simulink model "SSC"  (R2018b)
settings: Solver=ode23tb  StartTime=0.0  StopTime=5  RelTol=1e-3  EnableMultiTasking=on
values from neighbouring files (symbols this model uses):
  simSwitchingFrequency = 500.0    [SSC.sldd]
libraries: powerlib x15, powerlib_meascontrol x4, raspberrypilib x2, simulink x1, dspsrcs4 x1
settings Model: DataDictionary=SSC.sldd  SimulationMode=accelerator  Creator=guido  LastModifiedBy=guido
settings SolverCC: PositivePriorityOrder=on
settings OptimizationCC: EnhancedBackFolding=on  PassReuseOutputArgsAs=Individual arguments  EfficientMapNaN2IntZero=off  MaxStackSize=64  OptimizeBlockOrder=speed  DifferentSizesBufferReuse=on
settings DebuggingCC: ParameterTunabilityLossMsg=error
settings HardwareCC: ProdBitPerPointer=32  ProdBitPerSizeT=32  ProdBitPerPtrDiffT=32  ProdLargestAtomicInteger=Long  ProdLargestAtomicFloat=Double  ProdWordSize=32  ProdHWDeviceType=ARM Compatible->ARM Cortex  TargetBitPerPointer=64  TargetBitPerSizeT=64  TargetBitPerPtrDiffT=64  TargetLargestAtomicInteger=Long  TargetLongLongMode=on  TargetIntDivRoundTo=Zero  TargetEndianess=LittleEndian  TargetWordSize=64  TargetHWDeviceType=MATLAB Host  ProdEqTarget=off  UseEmbeddedCoderFeatures=off
settings SFSimCC: MATLABDynamicMemAlloc=off
settings CodeAppCC: MaxIdLength=128
settings GRTTargetCC: TargetLangStandard=C89/C90 (ANSI)  CombineOutputUpdateFcns=off  GRTInterface=on

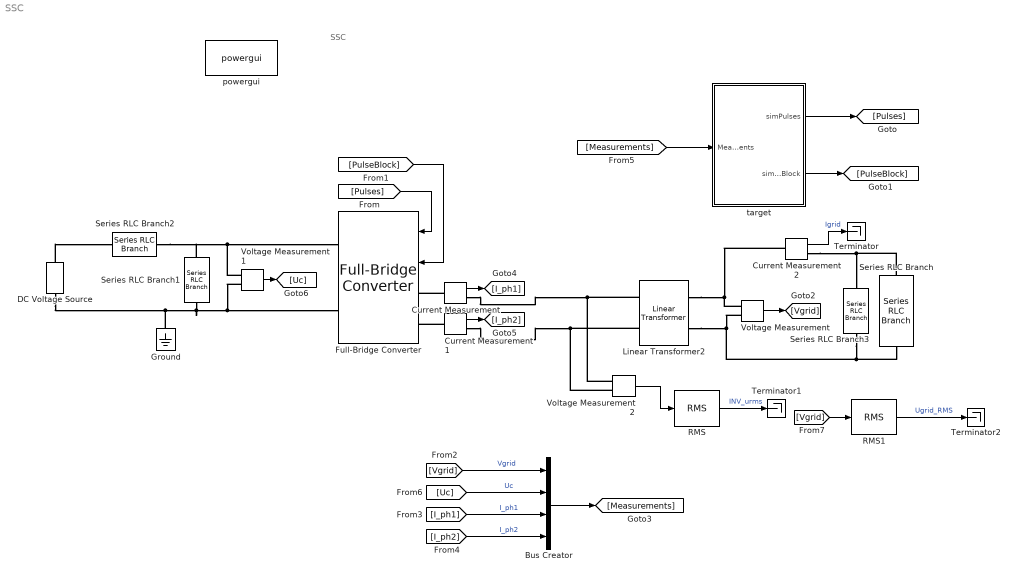
== system SSC ==
  note: SSC
  Bus Creator : BusCreator  Inputs=4  OutDataTypeStr=Bus: MeasurementsBus
  Current Measurement : powerlib/Measurements/Current Measurement  PhasorSimulation=off  OutputType=Complex  PSBequivalent=0
  Current Measurement1 : powerlib/Measurements/Current Measurement  PhasorSimulation=off  OutputType=Complex  PSBequivalent=0
  Current Measurement2 : powerlib/Measurements/Current Measurement  PhasorSimulation=off  OutputType=Complex  PSBequivalent=0
  DC Voltage Source : powerlib/Electrical Sources/DC Voltage Source  Amplitude=24  Measurements=None
  Full-Bridge Converter : powerlib/Power Electronics/Full-Bridge Converter  ModelType=Switching devices  Ron=1e-3  Rs=1e6  Cs=inf  Vforward=[0,0]  Ron_Diode=1e-3  Rs_Diode=1e6  Cs_Diode=inf  Vf_Diode=1e-3  Rs_CurrentSource=inf
      settings: SourceProductName=Simscape Power Systems  SourceProductBaseCode=PS
  Ground : powerlib/Elements/Ground  LConnTagsString=a
  Linear Transformer2 : powerlib/Elements/Linear Transformer  UNITS=pu  NominalPower=[ 1e3 50 ]  winding1="[ 12  0.002  0.08 ]"  winding2="[ 230  0.002  0.08 ]"  ThreeWindings=off  winding3=[ 315e3 0.002 0.08 ]  RmLm=[ 500 500 ]  Measurements=None  DataType=off
  RMS : powerlib_meascontrol/Measurements/RMS  TrueRMS=on  Freq=50  RMSInit=0  Ts=0
  RMS1 : powerlib_meascontrol/Measurements/RMS  TrueRMS=on  Freq=50  RMSInit=0  Ts=0
  Series RLC Branch : powerlib/Elements/Series RLC Branch  LConnTagsString=__new0  RConnTagsString=__new0  BranchType=RL  Resistance=10  Inductance=1  SetiL0=off  InitialCurrent=0  Capacitance=1e-6  Setx0=off  InitialVoltage=0  Measurements=None
  Series RLC Branch1 : powerlib/Elements/Series RLC Branch  LConnTagsString=__new0  RConnTagsString=__new0  BranchType=RC  Resistance=0.01  Inductance=1e-3  SetiL0=off  InitialCurrent=0  Capacitance=1e-3  Setx0=off  InitialVoltage=0  Measurements=None
  Series RLC Branch2 : powerlib/Elements/Series RLC Branch  LConnTagsString=__new0  RConnTagsString=__new0  BranchType=RL  Resistance=0.01  Inductance=1e-3  SetiL0=off  InitialCurrent=0  Capacitance=1e-3  Setx0=off  InitialVoltage=0  Measurements=None
  Series RLC Branch3 : powerlib/Elements/Series RLC Branch  LConnTagsString=__new0  RConnTagsString=__new0  BranchType=RC  Resistance=0.01  Inductance=1e-3  SetiL0=off  InitialCurrent=0  Capacitance=1e-4  Setx0=off  InitialVoltage=0  Measurements=None
  Terminator : Terminator
  Terminator1 : Terminator
  Terminator2 : Terminator
  Voltage Measurement : powerlib/Measurements/Voltage Measurement  PhasorSimulation=off  OutputType=Complex  PSBequivalent=0
  Voltage Measurement1 : powerlib/Measurements/Voltage Measurement  PhasorSimulation=off  OutputType=Complex  PSBequivalent=0
  Voltage Measurement2 : powerlib/Measurements/Voltage Measurement  PhasorSimulation=off  OutputType=Complex  PSBequivalent=0
  powergui : powerlib/powergui  Priority=1  SimulationMode=Discrete  SampleTime=50e-6  frequency=60  Iterations=50  frequencyindice=0  Pbase=100e6  ErrMax=1e-4  UnitsV=kV  UnitsW=MW  buscounter=0  FunctionMessages=off  echomessages=off  EnableUseOfTLC=off  CurrentSourceSwitches=off  DisableSnubberDevices=off  DisableRonSwitches=off  DisableVfSwitches=off  DisplayEquations=off  SolverType=Tustin/Backward Euler (TBE)  Interpol=off  ExternalGateDelay=off  methode=off  Ts=100  x0status=blocks  SPID=off  SwTol=0  HookPort=off  RestoreLinks=warning  ResistiveCurrentMeasurement=off  Frange=[0:2:500]  Ylog=off  Xlog=on  ShowGrid=off  save=off  variable=ZData  structure=0  ZoomFFT=off  StartTime=0.0  cycles=1  DisplayStyle=1  fundamental=60  FreqAxis=off  MaxFrequency=1000  frequencyindicesteady=1  RmsSteady=1  display=off
  target : Subsystem
      mask Display: disp('TARGET')
  wires:
  target/1(simPulses) -> [Pulses]
  [Pulses] -> Full-Bridge Converter/1
  target/2(simPulseBlock) -> [PulseBlock]
  [PulseBlock] -> Full-Bridge Converter/2
  [Measurements] -> target/1(Measurements)
  Voltage Measurement/1 -> [Vgrid]
  [Vgrid] -> Bus Creator/1  "Vgrid"
  Bus Creator/1 -> [Measurements]
  Current Measurement/1 -> [I_ph1]
  Current Measurement1/1 -> [I_ph2]
  [I_ph1] -> Bus Creator/3  "I_ph1"
  [I_ph2] -> Bus Creator/4  "I_ph2"
  Voltage Measurement1/1 -> [Uc]
  [Uc] -> Bus Creator/2  "Uc"
  Current Measurement2/1 -> Terminator/1  "Igrid"
  Voltage Measurement2/1 -> RMS/1
  RMS/1 -> Terminator1/1  "INV_urms"
  [Vgrid] -> RMS1/1
  RMS1/1 -> Terminator2/1  "Ugrid_RMS"
  connections:
  Voltage Measurement1/LConn1 -- Series RLC Branch2/LConn1 -- Series RLC Branch1/LConn1 -- Full-Bridge Converter/RConn1
  DC Voltage Source/LConn1 -- Ground/LConn1 -- Series RLC Branch1/RConn1 -- Full-Bridge Converter/RConn2 -- Voltage Measurement1/LConn2
  Current Measurement/LConn1 -- Full-Bridge Converter/LConn1
  Current Measurement2/RConn1 -- Series RLC Branch/LConn1 -- Series RLC Branch3/LConn1
  Current Measurement1/LConn1 -- Full-Bridge Converter/LConn2
  Series RLC Branch/RConn1 -- Series RLC Branch3/RConn1 -- Linear Transformer2/RConn2 -- Voltage Measurement/LConn2
  DC Voltage Source/RConn1 -- Series RLC Branch2/RConn1
  Current Measurement1/RConn1 -- Linear Transformer2/LConn2 -- Voltage Measurement2/LConn2
  Current Measurement/RConn1 -- Linear Transformer2/LConn1 -- Voltage Measurement2/LConn1
  Voltage Measurement/LConn1 -- Linear Transformer2/RConn1 -- Current Measurement2/LConn1

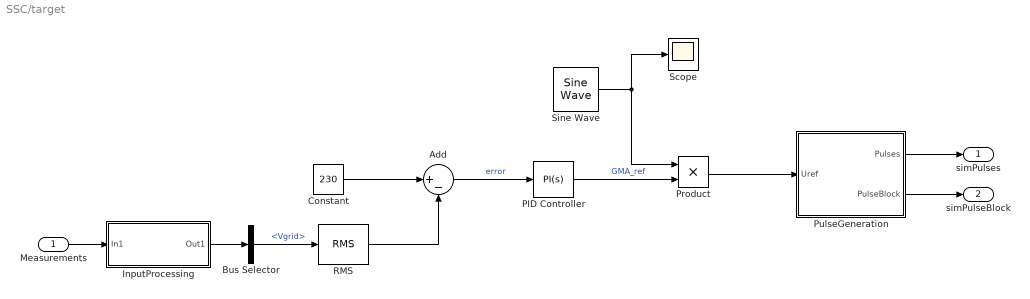
== system SSC/target ==
  Measurements : Inport
  Add : Sum  Inputs=|+-
  Bus Selector : BusSelector  OutputSignals=Vgrid
  Constant : Constant  Value=230
  InputProcessing : Subsystem
  PID Controller : simulink/Continuous/PID Controller  Controller=PI  Form=Parallel  TimeDomain=Continuous-time  SampleTime=-1  IntegratorMethod=Forward Euler  FilterMethod=Forward Euler  ControllerParametersSource=internal  P=1e-4  I=1e-2  D=0  UseFilter=on  N=100  TunerSelectOption=Transfer Function Based (PID Tuner App)  InitialConditionSource=internal  InitialConditionForIntegrator=0  InitialConditionForFilter=0  DifferentiatorICPrevScaledInput=0  ExternalReset=none  TrackingMode=off  Kt=1  LimitOutput=on  UpperSaturationLimit=1  LowerSaturationLimit=0  LinearizeAsGain=on  AntiWindupMode=clamping  Kb=1  POutMin=[]  POutMax=[]  IOutMin=[]  IOutMax=[]  DOutMin=[]  DOutMax=[]  NOutMin=[]  NOutMax=[]  SumOutMin=[]  SumOutMax=[]  SaturationOutMin=[]  SaturationOutMax=[]  PParamMin=[]  PParamMax=[]  IParamMin=[]  IParamMax=[]  DParamMin=[]  DParamMax=[]  NParamMin=[]  NParamMax=[]  KbParamMin=[]  KbParamMax=[]  KtParamMin=[]  KtParamMax=[]  KbOutMin=[]  KbOutMax=[]  KtOutMin=[]  KtOutMax=[]  IntegratorOutMin=[]  IntegratorOutMax=[]  FilterOutMin=[]  FilterOutMax=[]  SumI1OutMin=[]  SumI1OutMax=[]  SumI2OutMin=[]  SumI2OutMax=[]  SumI3OutMin=[]  SumI3OutMax=[]  SumI4OutMin=[]  SumI4OutMax=[]  SumDOutMin=[]  SumDOutMax=[]  DifferentiatorOutMin=[]  DifferentiatorOutMax=[]  FilterDiffOutCoefMin=[]  FilterDiffOutCoefMax=[]  ReciprocalOutMin=[]  ReciprocalOutMax=[]  SumDenOutMin=[]  SumDenOutMax=[]  SumNumOutMin=[]  SumNumOutMax=[]  DivideOutMin=[]  DivideOutMax=[]  IntegratorContinuousStateAttributes=''  IntegratorStateMustResolveToSignalObject=off  IntegratorRTWStateStorageClass=Auto  FilterContinuousStateAttributes=''  FilterStateMustResolveToSignalObject=off  FilterRTWStateStorageClass=Auto  ParallelPVariant=InternalParameters  IdealPVariant=Disabled  IVariant=InternalParameters  DVariant=Disabled  IntegratorVariant=Continuous  SatVariant=Enabled  AWVariant=ContClampingParallel  PCopyVariant=Disabled  TRVariant=Disabled  FdbkBlocksVariant=Forward  IdealPFdbkVariant=Disabled  SatFdbkVariant=Disabled  DerivativeFilterVariant=Disabled  NVariant=Disabled  NCopyVariant=Disabled_SignalSpec  FilterICVariant=Disabled  IntegratorICVariant=InternalICs  ExternalResetVariant=Disabled  TRSumVariant=Passthrough  SumFdbkVariant=Disabled  SumVariant=Sum_PI
  Product : Product
  PulseGeneration : Subsystem
  RMS : powerlib_meascontrol/Measurements/RMS  TrueRMS=off  Freq=50  RMSInit=0  Ts=0
  Scope : Scope
  Sine Wave : dspsrcs4/Sine Wave  Amplitude=1  Frequency=50  Phase=0  SampleMode=Discrete  OutComplex=Real  CompMethod=Trigonometric fcn  TableSize=Speed  SampleTime=1/(simSwitchingFrequency*2)  SamplesPerFrame=1  ResetState=Restart at time zero  OutputFrames=off  dataType=double  wordLen=16  udDataType=sfix(16)  fracBitsMode=Best precision  numFracBits=15  OutDataTypeStr=double  LastOutDataTypeStr=double
  simPulses : Outport
  simPulseBlock : Outport  Port=2
  wires:
  Measurements/1 -> InputProcessing/1(In1)
  PulseGeneration/1(Pulses) -> simPulses/1
  InputProcessing/1(Out1) -> Bus Selector/1
  PulseGeneration/2(PulseBlock) -> simPulseBlock/1
  Sine Wave/1 -> Product/1, Scope/1
  Product/1 -> PulseGeneration/1(Uref)
  Bus Selector/1 -> RMS/1  "<Vgrid>"
  PID Controller/1 -> Product/2  "GMA_ref"
  Add/1 -> PID Controller/1  "error"
  RMS/1 -> Add/2
  Constant/1 -> Add/1

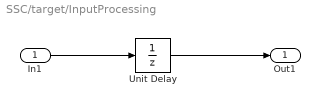
== system SSC/target/InputProcessing ==
  In1 : Inport
  Unit Delay : UnitDelay  SampleTime=-1
  Out1 : Outport
  wires:
  In1/1 -> Unit Delay/1
  Unit Delay/1 -> Out1/1

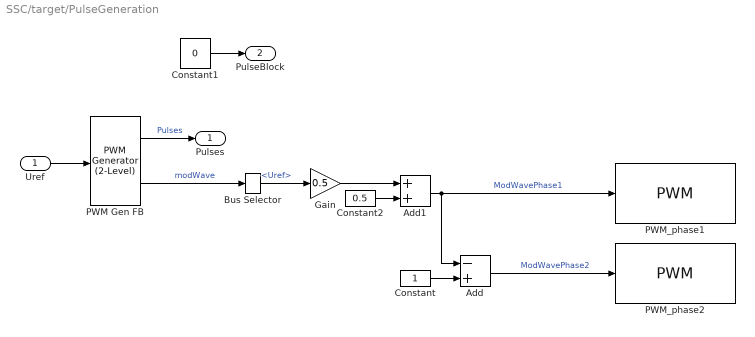
== system SSC/target/PulseGeneration ==
  Uref : Inport
  Add : Sum  Inputs=-+
  Add1 : Sum
  Bus Selector : BusSelector  OutputSignals=Uref
  Constant : Constant
  Constant1 : Constant  Value=0  OutDataTypeStr=boolean
  Constant2 : Constant  Value=0.5
  Gain : Gain  Gain=0.5
  PWM Gen FB : powerlib_meascontrol/Pulse & Signal Generators/PWM Generator (2-Level)  ModulatorType=Single-phase full-bridge (4 pulses)  ModulatorMode=Unsynchronized  Fc=simSwitchingFrequency  Pc=90  nF=27  MinMax="[ -1  1 ]"  SamplingTechnique=Symmetrical regular (single edge)  ModulatingSignals=off  m=0.8  Freq=60  Phase=0  Ts=1/(simSwitchingFrequency*10)  ShowCarrierOutport=on
  PWM_phase1 : raspberrypilib/PWM  board=Pi 2 Model B  Pin_=23  Frequency=8000  blockPlatform=Raspberry Pi
      settings: SourceProductName=Simulink Support Package for Raspberry Pi Hardware  SourceProductBaseCode=RASPPI
  PWM_phase2 : raspberrypilib/PWM  board=Pi 3 Model B  Pin_=24  Frequency=8000  blockPlatform=Raspberry Pi
      settings: SourceProductName=Simulink Support Package for Raspberry Pi Hardware  SourceProductBaseCode=RASPPI
  Pulses : Outport
  PulseBlock : Outport  Port=2
  wires:
  Uref/1 -> PWM Gen FB/1
  PWM Gen FB/1 -> Pulses/1  "Pulses"
  Bus Selector/1 -> Gain/1  "<Uref>"
  Add/1 -> PWM_phase2/1  "ModWavePhase2"
  Constant1/1 -> PulseBlock/1
  PWM Gen FB/2 -> Bus Selector/1  "modWave"
  Constant/1 -> Add/2
  Add1/1 -> Add/1, PWM_phase1/1  "ModWavePhase1"
  Gain/1 -> Add1/1
  Constant2/1 -> Add1/2
